simulink model "deposito_simu"  (R2023b)
settings: Solver=VariableStepAuto  StartTime=0.0  StopTime=300  RelTol=1e-3
values from neighbouring files (symbols this model uses):
  A = 15.52    [deposito.m]
  g = 981    [deposito.m]
settings Model: Creator=arlet  LastModifiedBy=arlet

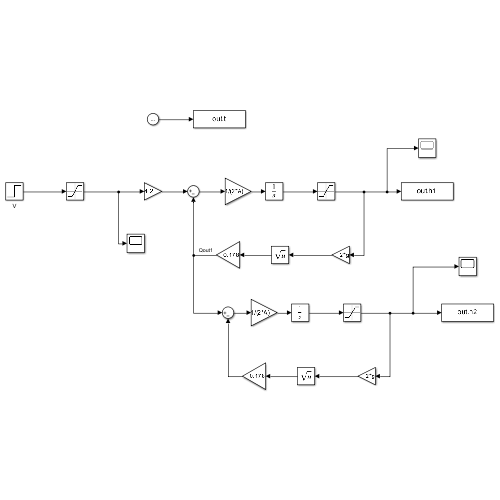
[thumbnail: Simulink's stored preview of the top-level diagram]
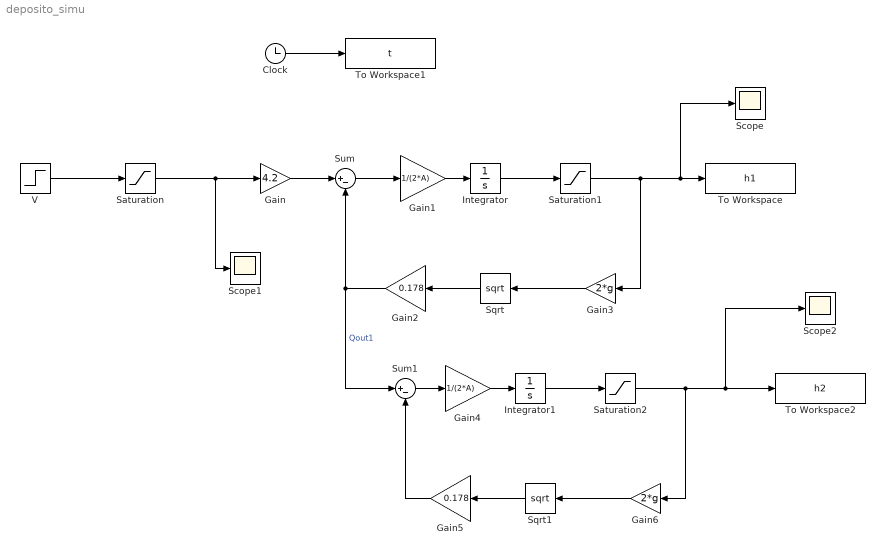
== system deposito_simu ==
  Clock : Clock
  Gain : Gain  Gain=4.2
  Gain1 : Gain  Gain=1/(2*A)
  Gain2 : Gain  Gain=0.178
  Gain3 : Gain  Gain=2*g
  Gain4 : Gain  Gain=1/(2*A)
  Gain5 : Gain  Gain=0.178
  Gain6 : Gain  Gain=2*g
  Integrator : Integrator
  Integrator1 : Integrator
  Saturation : Saturate  UpperLimit=20  LowerLimit=4
  Saturation1 : Saturate  UpperLimit=30  LowerLimit=0
  Saturation2 : Saturate  UpperLimit=30  LowerLimit=0
  Scope : Scope
  Scope1 : Scope
  Scope2 : Scope
  Sqrt : Sqrt
  Sqrt1 : Sqrt
  Sum : Sum  Inputs=|+-
  Sum1 : Sum  Inputs=|+-
  To Workspace : ToWorkspace  VariableName=h1  SaveFormat=Timeseries  SampleTime=-1
  To Workspace1 : ToWorkspace  VariableName=t  SaveFormat=Timeseries  SampleTime=-1
  To Workspace2 : ToWorkspace  VariableName=h2  SaveFormat=Timeseries  SampleTime=-1
  V : Step  Time=100  Before=6  After=8  SampleTime=0
  wires:
  Gain/1 -> Sum/1
  Integrator/1 -> Saturation1/1
  Gain1/1 -> Integrator/1
  Sum/1 -> Gain1/1
  V/1 -> Saturation/1
  Sqrt/1 -> Gain2/1
  Gain3/1 -> Sqrt/1
  Clock/1 -> To Workspace1/1
  Saturation/1 -> Scope1/1, Gain/1
  Saturation1/1 -> Gain3/1, Scope/1, To Workspace/1
  Saturation2/1 -> Gain6/1, To Workspace2/1, Scope2/1
  Sqrt1/1 -> Gain5/1
  Gain6/1 -> Sqrt1/1
  Gain5/1 -> Sum1/2
  Sum1/1 -> Gain4/1
  Gain2/1 -> Sum1/1, Sum/2  "Qout1"
  Integrator1/1 -> Saturation2/1
  Gain4/1 -> Integrator1/1
